simulink model "exampleModel"  (R2017b)
settings: Solver=VariableStepAuto  StartTime=0.0  StopTime=10e-6  RelTol=1e-3
PreLoadFcn:
  | setup
values from neighbouring files (symbols this model uses):
  axiClk = 156.25e6    (= 156250000)    [setup.m]    (also in setup_exampleModel_bus_axi_simulink.m; setup_exampleModel_bus_axi_simulink_lcls2.m; setup_lcls2_pcav.m)
  cav1p1_addr = 204    [setup_exampleModel_bus_axi_simulink.m]    (also in setup_exampleModel_bus_axi_simulink_lcls2.m; setup_lcls2_pcav.m; sysgen_signal.m)
  cav1p2_addr = cav1p1_addr * 2    (= 408)    [setup_exampleModel_bus_axi_simulink.m]    (also in setup_exampleModel_bus_axi_simulink_lcls2.m; setup_lcls2_pcav.m; sysgen_signal.m)
  cav2p1_addr = cav1p1_addr * 3    (= 612)    [setup_exampleModel_bus_axi_simulink.m]    (also in setup_exampleModel_bus_axi_simulink_lcls2.m; setup_lcls2_pcav.m; sysgen_signal.m)
  cav2p2_addr = cav1p1_addr * 4    (= 816)    [setup_exampleModel_bus_axi_simulink.m]    (also in setup_exampleModel_bus_axi_simulink_lcls2.m; setup_lcls2_pcav.m; sysgen_signal.m)
  Fadc = Fs/interleavedChannels    (= 29750000)    [setup.m]    (also in setup_exampleModel_bus_axi_simulink.m = 357000000; setup_exampleModel_bus_axi_simulink_lcls2.m = 351000000; setup_lcls2_pcav.m = 357000000)
  Fproc = 204e6    (= 204000000)    [setup_exampleModel_bus_axi_simulink.m]    (also in setup_exampleModel_bus_axi_simulink_lcls2.m = 200571400; setup_lcls2_pcav.m)
  Tadc = 1/fadc    (= 2.80112044818e-09)    [cavity_signal.m]    (also in setup_exampleModel_bus_axi_simulink.m; setup_exampleModel_bus_axi_simulink_lcls2.m = 2.849002849e-09; setup_lcls2_pcav.m; setup_pcav_simulink.m)
undefined symbols (not defined in the file or in its folder): AXI4, Lite
libraries: xbsIndex_r4 x248, llrf_lib x10, simulink x3
(part 3 of 3)

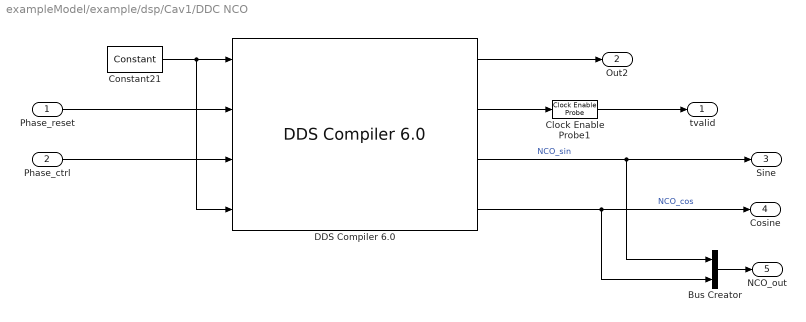
== system exampleModel/example/dsp/Cav1/DDC NCO ==
  Phase_reset : Inport
  Phase_ctrl : Inport  Port=2
  Bus Creator : BusCreator  Inputs=2
  Clock Enable Probe1 : xbsIndex_r4/Clock Enable Probe  inherit_constraints=on  block_type=ceprobe
      settings: infoedit="Clock enable extractor.  Produces a Boolean output that mirrors the hardware clock enable associated with the input sample rate.<br><br>Hardware notes: in hardware this block costs nothing."
  Constant21 : xbsIndex_r4/Constant  const=1  gui_display_data_type=Boolean  arith_type=Boolean  n_bits=4  bin_pt=0  preci_type=Single  exp_width=8  frac_width=24  explicit_period=off  period=1  equ=P=C  opselect=C  inp2=PCIN>>17  opr=+  inp1=P  carry=CIN  dbl_ovrd=off  block_type=constant
  "DDS Compiler 6.0 " : xbsIndex_r4/DDS Compiler 6.0   partspresent=Phase_Generator_and_SIN_COS_LUT  dds_clock_rate=Fproc*(1e-6)  channels=1  mode_of_operation=Standard  modulus=9  parameter_entry=System_Parameters  spurious_free_dynamic_range=60.00000000  frequency_resolution=0.40000000  noise_shaping=None  phase_width=29  output_width=10  output_selection=Sine_and_Cosine  negative_sine=off  negative_cosine=off  amplitude_mode=Unit_Circle  memory_type=Auto  optimization_goal=Auto  dsp48_use=Minimal  resync=on  latency_configuration=Auto  latency=1  has_phase_out=off  has_aclken=off  has_aresetn=off  explicit_period=on  period=1/Fproc  data_has_tlast=Not_Required  has_tready=on  s_phase_has_tuser=Not_Required  m_data_has_tuser=Not_Required  m_phase_has_tuser=Not_Required  s_phase_tuser_width=1  output_form=Twos_Complement  s_config_sync_mode=On_Vector  phase_increment=Streaming  output_frequency1=0  output_frequency2=0  output_frequency3=0  output_frequency4=0  output_frequency5=0  output_frequency6=0  output_frequency7=0  output_frequency8=0  output_frequency9=0  output_frequency10=0  output_frequency11=0  output_frequency12=0  output_frequency13=0  output_frequency14=0  output_frequency15=0  output_frequency16=0  pinc1='0'  pinc2='0'  pinc3='0'  pinc4='0'  pinc5='0'  pinc6='0'  pinc7='0'  pinc8='0'  pinc9='0'  pinc10='0'  pinc11='0'  pinc12='0'  pinc13='0'  pinc14='0'  pinc15='0'  pinc16='0'  phase_offset=None  phase_offset_angles1=0  phase_offset_angles2=0  phase_offset_angles3=0  phase_offset_angles4=0  phase_offset_angles5=0  phase_offset_angles6=0  phase_offset_angles7=0  phase_offset_angles8=0  phase_offset_angles9=0  phase_offset_angles10=0  phase_offset_angles11=0  phase_offset_angles12=0  phase_offset_angles13=0  phase_offset_angles14=0  phase_offset_angles15=0  phase_offset_angles16=0  poff1='0'  poff2='0'  poff3='0'  poff4='0'  poff5='0'  poff6='0'  poff7='0'  poff8='0'  poff9='0'  poff10='0'  poff11='0'  poff12='0'  poff13='0'  poff14='0'  poff15='0'  poff16='0'  trim_axipin_name=off  simulation_type=hybrid_sim  simulation_model=sysgen:xddsv6_0_cmodel  data_path_portlist={ 's_axis_config_tdata_poff', 's_axis_config_tdata_chan0_poff', 's_axis_config_tdata_pinc', 's_axis_config_tdata_chan0_pinc', 's_axis_phase_tdata_resync', 's_axis_phase_tdata_chan0_resync', 's_axis_phase_tdata_poff', 's_axis_phase_tdata_chan0_poff', 's_axis_phase_tdata_pinc', 's_axis_phase_tdata_chan0_pinc', 's_axis_phase_tdata_phase_in', 'm_axis_data_tdata_sine', 'm_axis_data_tdata_chan0_sine', 'm_axis_data_tdata_cosine', 'm_axis_data_tdata_chan0_cosine', 'm_axis_phase_tdata_phase_out', 'm_axis_phase_tdata_chan0_phase_out'}  por_mode=false  gui_behaviour=Sysgen  ip_name=DDS Compiler  ip_version=6.0  dsptool_ready=true  wrapper_available=true  port_translation_map={ 'aclken' => 'en', 'aresetn' => 'rst' }  ipcore_usecache=true  ipcore_useipmodelcache=true  ipcore_xco_need_fpga_part=true  ipcore_verbose=false  block_type=dds_compiler_v6_0
  tvalid : Outport
  Out2 : Outport  Port=2
  Sine : Outport  Port=3
  Cosine : Outport  Port=4
  NCO_out : Outport  Port=5
  wires:
  "DDS Compiler 6.0 "/1 -> Out2/1
  Constant21/1 -> "DDS Compiler 6.0 "/4, "DDS Compiler 6.0 "/1
  Clock Enable Probe1/1 -> tvalid/1
  "DDS Compiler 6.0 "/3 -> Bus Creator/1, Sine/1  "NCO_sin"
  "DDS Compiler 6.0 "/4 -> Bus Creator/2, Cosine/1  "NCO_cos"
  Phase_ctrl/1 -> "DDS Compiler 6.0 "/3
  Phase_reset/1 -> "DDS Compiler 6.0 "/2
  "DDS Compiler 6.0 "/2 -> Clock Enable Probe1/1
  Bus Creator/1 -> NCO_out/1

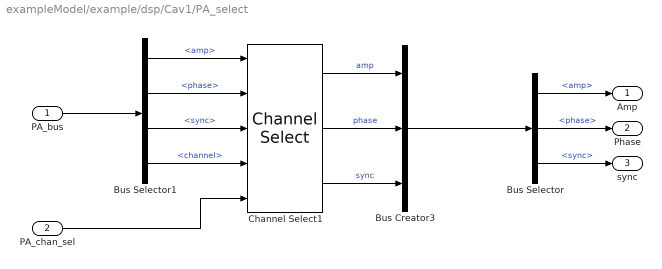
== system exampleModel/example/dsp/Cav1/PA_select ==
  PA_bus : Inport
  PA_chan_sel : Inport  Port=2
  Bus Creator3 : BusCreator  Inputs=3
  Bus Selector : BusSelector  OutputSignals=amp,phase,sync
  Bus Selector1 : BusSelector  OutputSignals=amp,phase,sync,channel
  Channel Select1 : llrf_lib/Sysgen/Single Rate/Channel Select  SystemSampleTime=-1
      settings: SourceProductName=LLRF Library
  Amp : Outport
  Phase : Outport  Port=2
  sync : Outport  Port=3
  wires:
  Bus Selector/3 -> sync/1  "<sync>"
  Bus Selector/2 -> Phase/1  "<phase>"
  Bus Selector/1 -> Amp/1  "<amp>"
  Bus Selector1/1 -> Channel Select1/1  "<amp>"
  Bus Selector1/2 -> Channel Select1/2  "<phase>"
  Bus Selector1/3 -> Channel Select1/3  "<sync>"
  Bus Selector1/4 -> Channel Select1/4  "<channel>"
  Channel Select1/1 -> Bus Creator3/1  "amp"
  Channel Select1/2 -> Bus Creator3/2  "phase"
  Channel Select1/3 -> Bus Creator3/3  "sync"
  Bus Creator3/1 -> Bus Selector/1
  PA_chan_sel/1 -> Channel Select1/5
  PA_bus/1 -> Bus Selector1/1

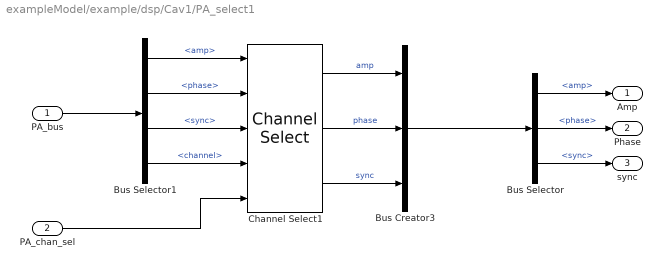
== system exampleModel/example/dsp/Cav1/PA_select1 ==
  PA_bus : Inport
  PA_chan_sel : Inport  Port=2
  Bus Creator3 : BusCreator  Inputs=3
  Bus Selector : BusSelector  OutputSignals=amp,phase,sync
  Bus Selector1 : BusSelector  OutputSignals=amp,phase,sync,channel
  Channel Select1 : llrf_lib/Sysgen/Single Rate/Channel Select  SystemSampleTime=-1
      settings: SourceProductName=LLRF Library
  Amp : Outport
  Phase : Outport  Port=2
  sync : Outport  Port=3
  wires:
  PA_bus/1 -> Bus Selector1/1
  PA_chan_sel/1 -> Channel Select1/5
  Bus Creator3/1 -> Bus Selector/1
  Channel Select1/3 -> Bus Creator3/3  "sync"
  Channel Select1/2 -> Bus Creator3/2  "phase"
  Channel Select1/1 -> Bus Creator3/1  "amp"
  Bus Selector1/4 -> Channel Select1/4  "<channel>"
  Bus Selector1/3 -> Channel Select1/3  "<sync>"
  Bus Selector1/2 -> Channel Select1/2  "<phase>"
  Bus Selector1/1 -> Channel Select1/1  "<amp>"
  Bus Selector/1 -> Amp/1  "<amp>"
  Bus Selector/2 -> Phase/1  "<phase>"
  Bus Selector/3 -> sync/1  "<sync>"

== system exampleModel/example/dsp/Cav1/Subsystem1 ==
  IQ_stream_in : Inport
  IQ_chan_sel : Inport  Port=2
  Bus Creator5 : BusCreator  Inputs=3
  Bus Selector : BusSelector  OutputSignals=ddcI,ddcQ,sync
  Bus Selector3 : BusSelector  OutputSignals=ddcI,ddcQ,ddcSync,ddcChannel
  Channel Select3 : llrf_lib/Sysgen/Single Rate/Channel Select  SystemSampleTime=-1
      settings: SourceProductName=LLRF Library
  ddcI : Outport
  ddcQ : Outport  Port=2
  sync : Outport  Port=3
  wires:
  IQ_stream_in/1 -> Bus Selector3/1
  IQ_chan_sel/1 -> Channel Select3/5
  Channel Select3/3 -> Bus Creator5/3  "sync"
  Bus Selector3/2 -> Channel Select3/2  "<ddcQ>"
  Channel Select3/1 -> Bus Creator5/1  "ddcI"
  Channel Select3/2 -> Bus Creator5/2  "ddcQ"
  Bus Selector3/1 -> Channel Select3/1  "<ddcI>"
  Bus Selector3/4 -> Channel Select3/4  "<ddcChannel>"
  Bus Selector3/3 -> Channel Select3/3  "<ddcSync>"
  Bus Creator5/1 -> Bus Selector/1
  Bus Selector/1 -> ddcI/1  "<ddcI>"
  Bus Selector/2 -> ddcQ/1  "<ddcQ>"
  Bus Selector/3 -> sync/1  "<sync>"

== system exampleModel/example/dsp/Cav1/Subsystem3 ==
  IQ_stream_in : Inport
  IQ_chan_sel : Inport  Port=2
  Bus Creator5 : BusCreator  Inputs=3
  Bus Selector : BusSelector  OutputSignals=ddcI,ddcQ,sync
  Bus Selector3 : BusSelector  OutputSignals=ddcI,ddcQ,ddcSync,ddcChannel
  Channel Select3 : llrf_lib/Sysgen/Single Rate/Channel Select  SystemSampleTime=-1
      settings: SourceProductName=LLRF Library
  ddcI : Outport
  ddcQ : Outport  Port=2
  sync : Outport  Port=3
  wires:
  Bus Selector/3 -> sync/1  "<sync>"
  Bus Selector/2 -> ddcQ/1  "<ddcQ>"
  Bus Selector/1 -> ddcI/1  "<ddcI>"
  Bus Creator5/1 -> Bus Selector/1
  Bus Selector3/3 -> Channel Select3/3  "<ddcSync>"
  Bus Selector3/4 -> Channel Select3/4  "<ddcChannel>"
  Bus Selector3/1 -> Channel Select3/1  "<ddcI>"
  Channel Select3/2 -> Bus Creator5/2  "ddcQ"
  Channel Select3/1 -> Bus Creator5/1  "ddcI"
  Bus Selector3/2 -> Channel Select3/2  "<ddcQ>"
  Channel Select3/3 -> Bus Creator5/3  "sync"
  IQ_chan_sel/1 -> Channel Select3/5
  IQ_stream_in/1 -> Bus Selector3/1

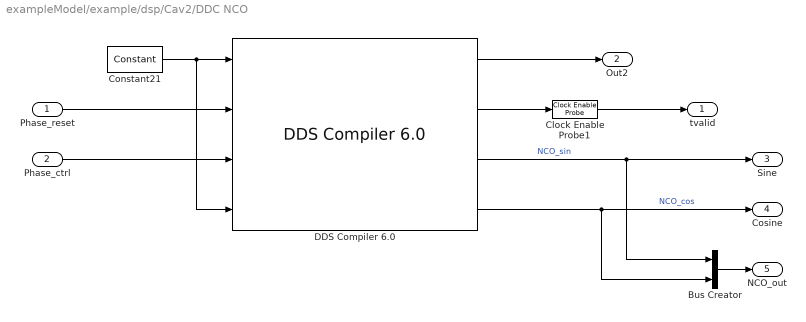
== system exampleModel/example/dsp/Cav2/DDC NCO ==
  Phase_reset : Inport
  Phase_ctrl : Inport  Port=2
  Bus Creator : BusCreator  Inputs=2
  Clock Enable Probe1 : xbsIndex_r4/Clock Enable Probe  inherit_constraints=on  block_type=ceprobe
      settings: infoedit="Clock enable extractor.  Produces a Boolean output that mirrors the hardware clock enable associated with the input sample rate.<br><br>Hardware notes: in hardware this block costs nothing."
  Constant21 : xbsIndex_r4/Constant  const=1  gui_display_data_type=Boolean  arith_type=Boolean  n_bits=4  bin_pt=0  preci_type=Single  exp_width=8  frac_width=24  explicit_period=off  period=1  equ=P=C  opselect=C  inp2=PCIN>>17  opr=+  inp1=P  carry=CIN  dbl_ovrd=off  block_type=constant
  "DDS Compiler 6.0 " : xbsIndex_r4/DDS Compiler 6.0   partspresent=Phase_Generator_and_SIN_COS_LUT  dds_clock_rate=Fproc*(1e-6)  channels=1  mode_of_operation=Standard  modulus=9  parameter_entry=System_Parameters  spurious_free_dynamic_range=60.00000000  frequency_resolution=0.40000000  noise_shaping=None  phase_width=29  output_width=10  output_selection=Sine_and_Cosine  negative_sine=off  negative_cosine=off  amplitude_mode=Unit_Circle  memory_type=Auto  optimization_goal=Auto  dsp48_use=Minimal  resync=on  latency_configuration=Auto  latency=1  has_phase_out=off  has_aclken=off  has_aresetn=off  explicit_period=on  period=1/Fproc  data_has_tlast=Not_Required  has_tready=on  s_phase_has_tuser=Not_Required  m_data_has_tuser=Not_Required  m_phase_has_tuser=Not_Required  s_phase_tuser_width=1  output_form=Twos_Complement  s_config_sync_mode=On_Vector  phase_increment=Streaming  output_frequency1=0  output_frequency2=0  output_frequency3=0  output_frequency4=0  output_frequency5=0  output_frequency6=0  output_frequency7=0  output_frequency8=0  output_frequency9=0  output_frequency10=0  output_frequency11=0  output_frequency12=0  output_frequency13=0  output_frequency14=0  output_frequency15=0  output_frequency16=0  pinc1='0'  pinc2='0'  pinc3='0'  pinc4='0'  pinc5='0'  pinc6='0'  pinc7='0'  pinc8='0'  pinc9='0'  pinc10='0'  pinc11='0'  pinc12='0'  pinc13='0'  pinc14='0'  pinc15='0'  pinc16='0'  phase_offset=None  phase_offset_angles1=0  phase_offset_angles2=0  phase_offset_angles3=0  phase_offset_angles4=0  phase_offset_angles5=0  phase_offset_angles6=0  phase_offset_angles7=0  phase_offset_angles8=0  phase_offset_angles9=0  phase_offset_angles10=0  phase_offset_angles11=0  phase_offset_angles12=0  phase_offset_angles13=0  phase_offset_angles14=0  phase_offset_angles15=0  phase_offset_angles16=0  poff1='0'  poff2='0'  poff3='0'  poff4='0'  poff5='0'  poff6='0'  poff7='0'  poff8='0'  poff9='0'  poff10='0'  poff11='0'  poff12='0'  poff13='0'  poff14='0'  poff15='0'  poff16='0'  trim_axipin_name=off  simulation_type=hybrid_sim  simulation_model=sysgen:xddsv6_0_cmodel  data_path_portlist={ 's_axis_config_tdata_poff', 's_axis_config_tdata_chan0_poff', 's_axis_config_tdata_pinc', 's_axis_config_tdata_chan0_pinc', 's_axis_phase_tdata_resync', 's_axis_phase_tdata_chan0_resync', 's_axis_phase_tdata_poff', 's_axis_phase_tdata_chan0_poff', 's_axis_phase_tdata_pinc', 's_axis_phase_tdata_chan0_pinc', 's_axis_phase_tdata_phase_in', 'm_axis_data_tdata_sine', 'm_axis_data_tdata_chan0_sine', 'm_axis_data_tdata_cosine', 'm_axis_data_tdata_chan0_cosine', 'm_axis_phase_tdata_phase_out', 'm_axis_phase_tdata_chan0_phase_out'}  por_mode=false  gui_behaviour=Sysgen  ip_name=DDS Compiler  ip_version=6.0  dsptool_ready=true  wrapper_available=true  port_translation_map={ 'aclken' => 'en', 'aresetn' => 'rst' }  ipcore_usecache=true  ipcore_useipmodelcache=true  ipcore_xco_need_fpga_part=true  ipcore_verbose=false  block_type=dds_compiler_v6_0
  tvalid : Outport
  Out2 : Outport  Port=2
  Sine : Outport  Port=3
  Cosine : Outport  Port=4
  NCO_out : Outport  Port=5
  wires:
  Bus Creator/1 -> NCO_out/1
  "DDS Compiler 6.0 "/2 -> Clock Enable Probe1/1
  Phase_reset/1 -> "DDS Compiler 6.0 "/2
  Phase_ctrl/1 -> "DDS Compiler 6.0 "/3
  "DDS Compiler 6.0 "/4 -> Cosine/1, Bus Creator/2  "NCO_cos"
  "DDS Compiler 6.0 "/3 -> Sine/1, Bus Creator/1  "NCO_sin"
  Clock Enable Probe1/1 -> tvalid/1
  Constant21/1 -> "DDS Compiler 6.0 "/1, "DDS Compiler 6.0 "/4
  "DDS Compiler 6.0 "/1 -> Out2/1

== system exampleModel/example/dsp/Cav2/PA_select ==
  PA_bus : Inport
  PA_chan_sel : Inport  Port=2
  Bus Creator3 : BusCreator  Inputs=3
  Bus Selector : BusSelector  OutputSignals=amp,phase,sync
  Bus Selector1 : BusSelector  OutputSignals=amp,phase,sync,channel
  Channel Select1 : llrf_lib/Sysgen/Single Rate/Channel Select  SystemSampleTime=-1
      settings: SourceProductName=LLRF Library
  Amp : Outport
  Phase : Outport  Port=2
  sync : Outport  Port=3
  wires:
  PA_bus/1 -> Bus Selector1/1
  PA_chan_sel/1 -> Channel Select1/5
  Bus Creator3/1 -> Bus Selector/1
  Channel Select1/3 -> Bus Creator3/3  "sync"
  Channel Select1/2 -> Bus Creator3/2  "phase"
  Channel Select1/1 -> Bus Creator3/1  "amp"
  Bus Selector1/4 -> Channel Select1/4  "<channel>"
  Bus Selector1/3 -> Channel Select1/3  "<sync>"
  Bus Selector1/2 -> Channel Select1/2  "<phase>"
  Bus Selector1/1 -> Channel Select1/1  "<amp>"
  Bus Selector/1 -> Amp/1  "<amp>"
  Bus Selector/2 -> Phase/1  "<phase>"
  Bus Selector/3 -> sync/1  "<sync>"

== system exampleModel/example/dsp/Cav2/PA_select1 ==
  PA_bus : Inport
  PA_chan_sel : Inport  Port=2
  Bus Creator3 : BusCreator  Inputs=3
  Bus Selector : BusSelector  OutputSignals=amp,phase,sync
  Bus Selector1 : BusSelector  OutputSignals=amp,phase,sync,channel
  Channel Select1 : llrf_lib/Sysgen/Single Rate/Channel Select  SystemSampleTime=-1
      settings: SourceProductName=LLRF Library
  Amp : Outport
  Phase : Outport  Port=2
  sync : Outport  Port=3
  wires:
  Bus Selector/3 -> sync/1  "<sync>"
  Bus Selector/2 -> Phase/1  "<phase>"
  Bus Selector/1 -> Amp/1  "<amp>"
  Bus Selector1/1 -> Channel Select1/1  "<amp>"
  Bus Selector1/2 -> Channel Select1/2  "<phase>"
  Bus Selector1/3 -> Channel Select1/3  "<sync>"
  Bus Selector1/4 -> Channel Select1/4  "<channel>"
  Channel Select1/1 -> Bus Creator3/1  "amp"
  Channel Select1/2 -> Bus Creator3/2  "phase"
  Channel Select1/3 -> Bus Creator3/3  "sync"
  Bus Creator3/1 -> Bus Selector/1
  PA_chan_sel/1 -> Channel Select1/5
  PA_bus/1 -> Bus Selector1/1

== system exampleModel/example/dsp/Cav2/Subsystem1 ==
  IQ_stream_in : Inport
  IQ_chan_sel : Inport  Port=2
  Bus Creator5 : BusCreator  Inputs=3
  Bus Selector : BusSelector  OutputSignals=ddcI,ddcQ,sync
  Bus Selector3 : BusSelector  OutputSignals=ddcI,ddcQ,ddcSync,ddcChannel
  Channel Select3 : llrf_lib/Sysgen/Single Rate/Channel Select  SystemSampleTime=-1
      settings: SourceProductName=LLRF Library
  ddcI : Outport
  ddcQ : Outport  Port=2
  sync : Outport  Port=3
  wires:
  Bus Selector/3 -> sync/1  "<sync>"
  Bus Selector/2 -> ddcQ/1  "<ddcQ>"
  Bus Selector/1 -> ddcI/1  "<ddcI>"
  Bus Creator5/1 -> Bus Selector/1
  Bus Selector3/3 -> Channel Select3/3  "<ddcSync>"
  Bus Selector3/4 -> Channel Select3/4  "<ddcChannel>"
  Bus Selector3/1 -> Channel Select3/1  "<ddcI>"
  Channel Select3/2 -> Bus Creator5/2  "ddcQ"
  Channel Select3/1 -> Bus Creator5/1  "ddcI"
  Bus Selector3/2 -> Channel Select3/2  "<ddcQ>"
  Channel Select3/3 -> Bus Creator5/3  "sync"
  IQ_chan_sel/1 -> Channel Select3/5
  IQ_stream_in/1 -> Bus Selector3/1

== system exampleModel/example/dsp/Cav2/Subsystem3 ==
  IQ_stream_in : Inport
  IQ_chan_sel : Inport  Port=2
  Bus Creator5 : BusCreator  Inputs=3
  Bus Selector : BusSelector  OutputSignals=ddcI,ddcQ,sync
  Bus Selector3 : BusSelector  OutputSignals=ddcI,ddcQ,ddcSync,ddcChannel
  Channel Select3 : llrf_lib/Sysgen/Single Rate/Channel Select  SystemSampleTime=-1
      settings: SourceProductName=LLRF Library
  ddcI : Outport
  ddcQ : Outport  Port=2
  sync : Outport  Port=3
  wires:
  IQ_stream_in/1 -> Bus Selector3/1
  IQ_chan_sel/1 -> Channel Select3/5
  Channel Select3/3 -> Bus Creator5/3  "sync"
  Bus Selector3/2 -> Channel Select3/2  "<ddcQ>"
  Channel Select3/1 -> Bus Creator5/1  "ddcI"
  Channel Select3/2 -> Bus Creator5/2  "ddcQ"
  Bus Selector3/1 -> Channel Select3/1  "<ddcI>"
  Bus Selector3/4 -> Channel Select3/4  "<ddcChannel>"
  Bus Selector3/3 -> Channel Select3/3  "<ddcSync>"
  Bus Creator5/1 -> Bus Selector/1
  Bus Selector/1 -> ddcI/1  "<ddcI>"
  Bus Selector/2 -> ddcQ/1  "<ddcQ>"
  Bus Selector/3 -> sync/1  "<sync>"

== system exampleModel/example/dsp/Ref/IQ_select ==
  IQ_stream_in : Inport
  IQ_chan_sel : Inport  Port=2
  Bus Creator5 : BusCreator  Inputs=3
  Bus Selector : BusSelector  OutputSignals=ddcI,ddcQ,sync
  Bus Selector3 : BusSelector  OutputSignals=ddcI,ddcQ,ddcSync,ddcChannel
  Channel Select3 : llrf_lib/Sysgen/Single Rate/Channel Select  SystemSampleTime=-1
      settings: SourceProductName=LLRF Library
  ddcI : Outport
  ddcQ : Outport  Port=2
  sync : Outport  Port=3
  wires:
  IQ_stream_in/1 -> Bus Selector3/1
  IQ_chan_sel/1 -> Channel Select3/5
  Channel Select3/3 -> Bus Creator5/3  "sync"
  Bus Selector3/2 -> Channel Select3/2  "<ddcQ>"
  Channel Select3/1 -> Bus Creator5/1  "ddcI"
  Channel Select3/2 -> Bus Creator5/2  "ddcQ"
  Bus Selector3/1 -> Channel Select3/1  "<ddcI>"
  Bus Selector3/4 -> Channel Select3/4  "<ddcChannel>"
  Bus Selector3/3 -> Channel Select3/3  "<ddcSync>"
  Bus Creator5/1 -> Bus Selector/1
  Bus Selector/1 -> ddcI/1  "<ddcI>"
  Bus Selector/2 -> ddcQ/1  "<ddcQ>"
  Bus Selector/3 -> sync/1  "<sync>"

== system exampleModel/example/dsp/Ref/PA_select ==
  PA_bus : Inport
  PA_chan_sel : Inport  Port=2
  Bus Creator3 : BusCreator  Inputs=3
  Bus Selector : BusSelector  OutputSignals=amp,phase,sync
  Bus Selector1 : BusSelector  OutputSignals=amp,phase,sync,channel
  Channel Select1 : llrf_lib/Sysgen/Single Rate/Channel Select  SystemSampleTime=-1
      settings: SourceProductName=LLRF Library
  Amp : Outport
  Phase : Outport  Port=2
  sync : Outport  Port=3
  wires:
  PA_bus/1 -> Bus Selector1/1
  PA_chan_sel/1 -> Channel Select1/5
  Bus Creator3/1 -> Bus Selector/1
  Channel Select1/3 -> Bus Creator3/3  "sync"
  Channel Select1/2 -> Bus Creator3/2  "phase"
  Channel Select1/1 -> Bus Creator3/1  "amp"
  Bus Selector1/4 -> Channel Select1/4  "<channel>"
  Bus Selector1/3 -> Channel Select1/3  "<sync>"
  Bus Selector1/2 -> Channel Select1/2  "<phase>"
  Bus Selector1/1 -> Channel Select1/1  "<amp>"
  Bus Selector/1 -> Amp/1  "<amp>"
  Bus Selector/2 -> Phase/1  "<phase>"
  Bus Selector/3 -> sync/1  "<sync>"
